simulink model "Bus_Mux"  (Simulink 8.0)
settings: Solver=ode45  StartTime=0.0  StopTime=10.0  RelTol=1e-3
settings Model: Creator=Faradars  LastModifiedBy=Faradars

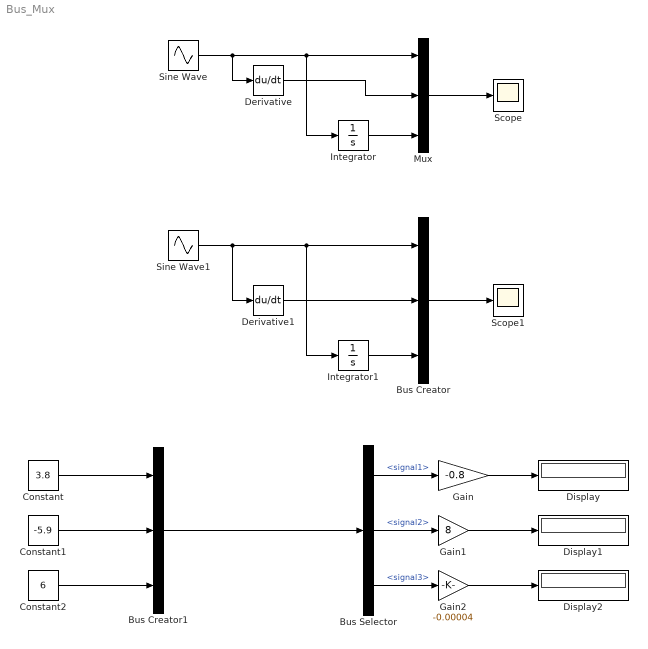
== system Bus_Mux ==
  Bus Creator : BusCreator  Inputs=3
  Bus Creator1 : BusCreator  Inputs=3
  Bus Selector : BusSelector
  Constant : Constant  Value=3.8
  Constant1 : Constant  Value=-5.9
  Constant2 : Constant  Value=6
  Derivative : Derivative
  Derivative1 : Derivative
  Display : Display
  Display1 : Display
  Display2 : Display
  Gain : Gain  Gain=-0.8
  Gain1 : Gain  Gain=8
  Gain2 : Gain  Gain=-0.00004
  Integrator : Integrator
  Integrator1 : Integrator
  Mux : Mux  Inputs=3
  Scope : Scope
  Scope1 : Scope
  Sine Wave : Sin  Amplitude=2  SampleTime=0
  Sine Wave1 : Sin  Amplitude=2  SampleTime=0
  wires:
  Sine Wave/1 -> Derivative/1, Integrator/1, Mux/1
  Derivative/1 -> Mux/2
  Integrator/1 -> Mux/3
  Mux/1 -> Scope/1
  Sine Wave1/1 -> Derivative1/1, Bus Creator/1, Integrator1/1
  Derivative1/1 -> Bus Creator/2
  Integrator1/1 -> Bus Creator/3
  Bus Creator/1 -> Scope1/1
  Bus Creator1/1 -> Bus Selector/1
  Bus Selector/1 -> Gain/1  "<signal1>"
  Gain/1 -> Display/1
  Bus Selector/2 -> Gain1/1  "<signal2>"
  Gain1/1 -> Display1/1
  Gain2/1 -> Display2/1
  Bus Selector/3 -> Gain2/1  "<signal3>"
  Constant/1 -> Bus Creator1/1
  Constant2/1 -> Bus Creator1/3
  Constant1/1 -> Bus Creator1/2
